simulink model "pid_test"  (R2021b)
settings: Solver=VariableStepAuto  StartTime=0.0  StopTime=3.0  RelTol=1e-3
settings Model: Creator=duanlinding  LastModifiedBy=duanlinding
settings DebuggingCC: AlgebraicLoopMsg=none

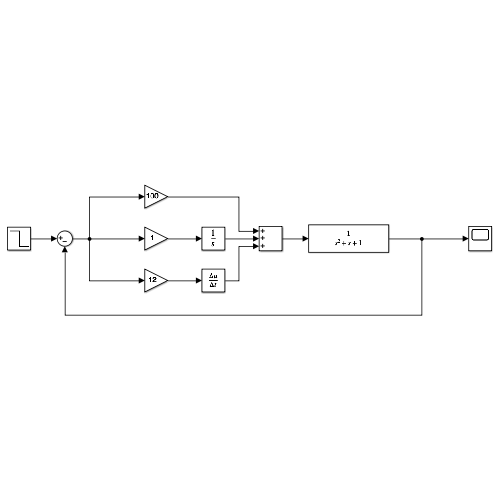
[thumbnail: Simulink's stored preview of the top-level diagram]
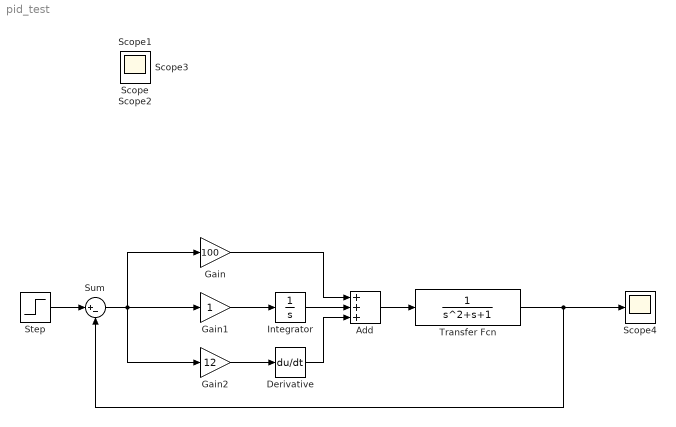
== system pid_test ==
  Add : Sum  Inputs=+++
  Derivative : Derivative
  Gain : Gain  Gain=100
  Gain1 : Gain
  Gain2 : Gain  Gain=12
  Integrator : Integrator
  Scope{,1..4} (5 alike) : Scope
  Step : Step  Before=10  After=5  SampleTime=0
  Sum : Sum  Inputs=|+-
  Transfer Fcn : TransferFcn  Denominator=[1 1 1]
  wires:
  Step/1 -> Sum/1
  Sum/1 -> Gain/1, Gain1/1, Gain2/1
  Gain/1 -> Add/1
  Integrator/1 -> Add/2
  Derivative/1 -> Add/3
  Gain1/1 -> Integrator/1
  Gain2/1 -> Derivative/1
  Transfer Fcn/1 -> Sum/2, Scope4/1
  Add/1 -> Transfer Fcn/1
